simulink model "STFTDiffWindowSizes"  (R2021b)
settings: Solver=VariableStepAuto  StartTime=0.0  StopTime=2048*15/fs  RelTol=1e-3
InitFcn:
  | f = 12.288e6;
  | fs = 153.6e6;
  | N1 = 256;
  | N2 = 512;
  | N3 = 1024;
  | N4 = 2048;
  | N5 = 4096;
  | n1 = 0:N1-1;
  | n2 = 0:N2-1;
  | n3 = 0:N3-1;
  | n4 = 0:N4-1;
  | n5 = 0:N5-1;
  | Hamming1 = 0.54 - 0.46 * cos(2*pi*n1/N1);
  | Hamming2 = 0.54 - 0.46 * cos(2*pi*n2/N2);
  | Hamming3 = 0.54 - 0.46 * cos(2*pi*n3/N3);
  | Hamming4 = 0.54 - 0.46 * cos(2*pi*n4/N4);
  | Hamming5 = 0.54 - 0.46 * cos(2*pi*n5/N5);
  | Hanning1 = 0.5 * (1 + cos(2*pi*n1/N1));
  | Hanning2 = 0.5 * (1 + cos(2*pi*n2/N2));
  | Hanning3 = 0.5 * (1 + cos(2*pi*n3/N3));
  | Hanning4 = 0.5 * (1 + cos(2*pi*n4/N4));
  | Hanning5 = 0.5 * (1 + cos(2*pi*n5/N5));
  | Norm_Ham1 = sum(Hamming1);
  | Norm_Ham2 = sum(Hamming2);
  | Norm_Ham3 = sum(Hamming3);
  | Norm_Ham4 = sum(Hamming4);
  | Norm_Ham5 = sum(Hamming5);
  | Norm_Han1 = sum(Hanning1);
  | Norm_Han2 = sum(Hanning2);
  | Norm_Han3 = sum(Hanning3);
  | Norm_Han4 = sum(Hanning4);
  | Norm_Han5 = sum(Hanning5);
undefined symbols (not defined in the file): AXI4, Lite, Norm_Ham, Norm_Han
libraries: hdlBasic x321, hdlDSPIP x10, hdlsllib x1, vmcUtilities x1
(part 1 of 3)
settings Model: Creator=yxb20126  LastModifiedBy=yxb20126

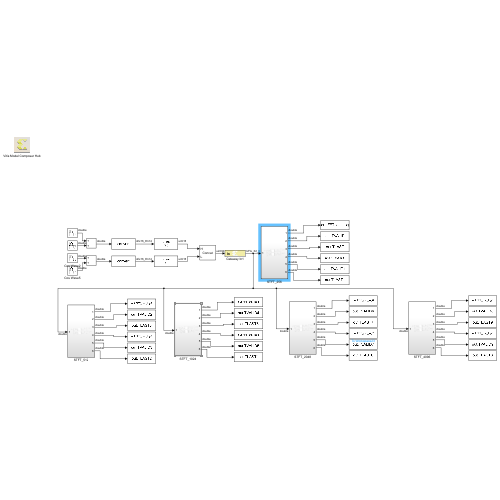
[thumbnail: Simulink's stored preview of the top-level diagram]
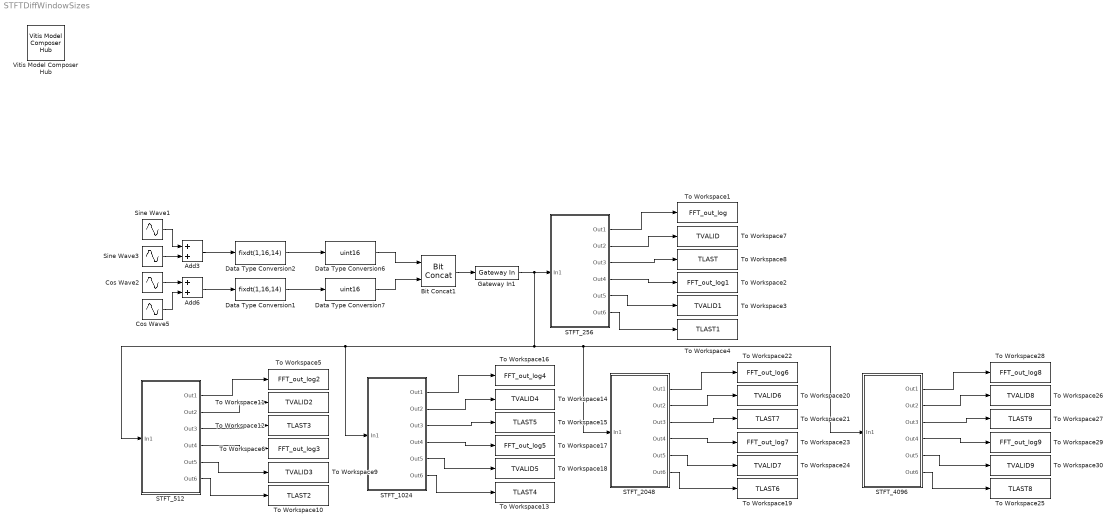
== system STFTDiffWindowSizes ==
  Add3 : Sum
  Add6 : Sum
  Bit Concat1 : hdlsllib/Logic and Bit Operations/Bit Concat  numInputs=2
  Cos Wave2 : Sin  Frequency=f*2*pi  Phase=pi/2  SampleTime=1/fs
  Cos Wave5 : Sin  Frequency=f*pi  Phase=pi/2  SampleTime=1/fs
  Data Type Conversion1 : DataTypeConversion  OutDataTypeStr=fixdt(1,16,14)  SaturateOnIntegerOverflow=on
  Data Type Conversion2 : DataTypeConversion  OutDataTypeStr=fixdt(1,16,14)  SaturateOnIntegerOverflow=on
  Data Type Conversion6 : DataTypeConversion  OutDataTypeStr=uint16  ConvertRealWorld=Stored Integer (SI)
  Data Type Conversion7 : DataTypeConversion  OutDataTypeStr=uint16  ConvertRealWorld=Stored Integer (SI)
  Gateway In1 : hdlBasic/Gateway In  gui_display_data_type=Fixed-point  arith_type=Unsigned  n_bits=32  bin_pt=0  preci_type=Single  exp_width=8  frac_width=24  rows=1  columns=1  quantization="Round  (unbiased: +/- Inf)"  overflow=Saturate  period=1/fs  UseAsADC=off  ADCChannel='1'  interface=None  automatic_assignment=on  address_offset=hex2dec('00')  intf_name=''  intf_description=''  default_value=0  timing_constraint=None  locs_specified=off  LOCs={}  io_standard={}  inherit_from_input=off  hdl_port=on  XmcBlockStatus=1  maskContainerNames=group4  block_type=gatewayin  block_config=sysgen:gateway_in_config  block_width_w=590  block_height_w=620  block_width=640  block_height=850
  STFT_1024 : Subsystem
  STFT_2048 : Subsystem
  STFT_256 : Subsystem
  STFT_4096 : Subsystem
  STFT_512 : Subsystem
  Sine Wave1 : Sin  Frequency=f*2*pi  SampleTime=1/fs
  Sine Wave3 : Sin  Frequency=f*pi  SampleTime=1/fs
  To Workspace1 : ToWorkspace  VariableName=FFT_out_log  SampleTime=-1
      settings: Save2DSignal=2-D array (concatenate along first dimension)
  To Workspace10 : ToWorkspace  VariableName=TLAST2  SampleTime=1/fs
      settings: Save2DSignal=2-D array (concatenate along first dimension)
  To Workspace11 : ToWorkspace  VariableName=TVALID2  SampleTime=1/fs
      settings: Save2DSignal=2-D array (concatenate along first dimension)
  To Workspace12 : ToWorkspace  VariableName=TLAST3  SampleTime=1/fs
      settings: Save2DSignal=2-D array (concatenate along first dimension)
  To Workspace13 : ToWorkspace  VariableName=TLAST4  SampleTime=1/fs
      settings: Save2DSignal=2-D array (concatenate along first dimension)
  To Workspace14 : ToWorkspace  VariableName=TVALID4  SampleTime=1/fs
      settings: Save2DSignal=2-D array (concatenate along first dimension)
  To Workspace15 : ToWorkspace  VariableName=TLAST5  SampleTime=1/fs
      settings: Save2DSignal=2-D array (concatenate along first dimension)
  To Workspace16 : ToWorkspace  VariableName=FFT_out_log4  SampleTime=-1
      settings: Save2DSignal=2-D array (concatenate along first dimension)
  To Workspace17 : ToWorkspace  VariableName=FFT_out_log5  SampleTime=-1
      settings: Save2DSignal=2-D array (concatenate along first dimension)
  To Workspace18 : ToWorkspace  VariableName=TVALID5  SampleTime=1/fs
      settings: Save2DSignal=2-D array (concatenate along first dimension)
  To Workspace19 : ToWorkspace  VariableName=TLAST6  SampleTime=1/fs
      settings: Save2DSignal=2-D array (concatenate along first dimension)
  To Workspace2 : ToWorkspace  VariableName=FFT_out_log1  SampleTime=-1
      settings: Save2DSignal=2-D array (concatenate along first dimension)
  To Workspace20 : ToWorkspace  VariableName=TVALID6  SampleTime=1/fs
      settings: Save2DSignal=2-D array (concatenate along first dimension)
  To Workspace21 : ToWorkspace  VariableName=TLAST7  SampleTime=1/fs
      settings: Save2DSignal=2-D array (concatenate along first dimension)
  To Workspace22 : ToWorkspace  VariableName=FFT_out_log6  SampleTime=-1
      settings: Save2DSignal=2-D array (concatenate along first dimension)
  To Workspace23 : ToWorkspace  VariableName=FFT_out_log7  SampleTime=-1
      settings: Save2DSignal=2-D array (concatenate along first dimension)
  To Workspace24 : ToWorkspace  VariableName=TVALID7  SampleTime=1/fs
      settings: Save2DSignal=2-D array (concatenate along first dimension)
  To Workspace25 : ToWorkspace  VariableName=TLAST8  SampleTime=1/fs
      settings: Save2DSignal=2-D array (concatenate along first dimension)
  To Workspace26 : ToWorkspace  VariableName=TVALID8  SampleTime=1/fs
      settings: Save2DSignal=2-D array (concatenate along first dimension)
  To Workspace27 : ToWorkspace  VariableName=TLAST9  SampleTime=1/fs
      settings: Save2DSignal=2-D array (concatenate along first dimension)
  To Workspace28 : ToWorkspace  VariableName=FFT_out_log8  SampleTime=-1
      settings: Save2DSignal=2-D array (concatenate along first dimension)
  To Workspace29 : ToWorkspace  VariableName=FFT_out_log9  SampleTime=-1
      settings: Save2DSignal=2-D array (concatenate along first dimension)
  To Workspace3 : ToWorkspace  VariableName=TVALID1  SampleTime=1/fs
      settings: Save2DSignal=2-D array (concatenate along first dimension)
  To Workspace30 : ToWorkspace  VariableName=TVALID9  SampleTime=1/fs
      settings: Save2DSignal=2-D array (concatenate along first dimension)
  To Workspace4 : ToWorkspace  VariableName=TLAST1  SampleTime=1/fs
      settings: Save2DSignal=2-D array (concatenate along first dimension)
  To Workspace5 : ToWorkspace  VariableName=FFT_out_log2  SampleTime=-1
      settings: Save2DSignal=2-D array (concatenate along first dimension)
  To Workspace6 : ToWorkspace  VariableName=FFT_out_log3  SampleTime=-1
      settings: Save2DSignal=2-D array (concatenate along first dimension)
  To Workspace7 : ToWorkspace  VariableName=TVALID  SampleTime=1/fs
      settings: Save2DSignal=2-D array (concatenate along first dimension)
  To Workspace8 : ToWorkspace  VariableName=TLAST  SampleTime=1/fs
      settings: Save2DSignal=2-D array (concatenate along first dimension)
  To Workspace9 : ToWorkspace  VariableName=TVALID3  SampleTime=1/fs
      settings: Save2DSignal=2-D array (concatenate along first dimension)
  Vitis Model Composer Hub : vmcUtilities/Vitis Model Composer Hub  Tag=genX  CodeGeneration=off  SubsystemName=<enter or select subsystem name>  TargetDirectory=./code  ExportType=HLS C++ code  IpVendor=xilinx.com  IpLibrary=hls  IpVersion=1.0  IpHWLanguage=Verilog  AieCompilerOptions={}  CreateTestbench=off  TestbenchStackSize=10  RunAieSim=off  AieSimTimeout=50000  RunAieSimProfiling=off  LaunchVitisAnalyzer=off  PlotOutput=off  RunX86Sim=off  X86SimTimeout=10  GenHwImage=off  PlatformType=Not Specified  HwSystemType=Baremetal  HwValidationTarget=hw  ProjDevice=xczu48dr-ffvg1517-2-e  ProjDevicePart=xczu48dr-ffvg1517-2-e  SamplePeriod=-1  ClockFrequency=200  DataPathParallelism=1  xilinxfamily=zynquplusRFSOC  part=xczu48dr  speed=-2-e  package=ffvg1517  directory=./netlist  testbench=off  incr_netlist=off  synthesis_tool=Vivado  clock_wrapper=Clock Enables  dbl_ovrd=According to Block Masks  dcm_input_clock_period=10  sysclk_period=(1/fs)*10e9  simulink_period=1/fs  eval_field=0
  wires:
  Data Type Conversion1/1 -> Data Type Conversion7/1
  Data Type Conversion2/1 -> Data Type Conversion6/1
  Data Type Conversion6/1 -> Bit Concat1/1
  Bit Concat1/1 -> Gateway In1/1
  Add3/1 -> Data Type Conversion2/1
  Add6/1 -> Data Type Conversion1/1
  Data Type Conversion7/1 -> Bit Concat1/2
  Gateway In1/1 -> STFT_1024/1(In1), STFT_512/1(In1), STFT_2048/1(In1), STFT_4096/1(In1), STFT_256/1(In1)
  Cos Wave2/1 -> Add6/1
  Sine Wave1/1 -> Add3/1
  Cos Wave5/1 -> Add6/2
  Sine Wave3/1 -> Add3/2
  STFT_256/1(Out1) -> To Workspace1/1
  STFT_256/2(Out2) -> To Workspace7/1
  STFT_256/3(Out3) -> To Workspace8/1
  STFT_256/4(Out4) -> To Workspace2/1
  STFT_256/5(Out5) -> To Workspace3/1
  STFT_256/6(Out6) -> To Workspace4/1
  STFT_512/6(Out6) -> To Workspace10/1
  STFT_512/5(Out5) -> To Workspace9/1
  STFT_512/4(Out4) -> To Workspace6/1
  STFT_512/3(Out3) -> To Workspace12/1
  STFT_512/2(Out2) -> To Workspace11/1
  STFT_512/1(Out1) -> To Workspace5/1
  STFT_1024/1(Out1) -> To Workspace16/1
  STFT_1024/2(Out2) -> To Workspace14/1
  STFT_1024/3(Out3) -> To Workspace15/1
  STFT_1024/4(Out4) -> To Workspace17/1
  STFT_1024/5(Out5) -> To Workspace18/1
  STFT_1024/6(Out6) -> To Workspace13/1
  STFT_2048/6(Out6) -> To Workspace19/1
  STFT_2048/5(Out5) -> To Workspace24/1
  STFT_2048/4(Out4) -> To Workspace23/1
  STFT_2048/3(Out3) -> To Workspace21/1
  STFT_2048/2(Out2) -> To Workspace20/1
  STFT_2048/1(Out1) -> To Workspace22/1
  STFT_4096/1(Out1) -> To Workspace28/1
  STFT_4096/2(Out2) -> To Workspace26/1
  STFT_4096/3(Out3) -> To Workspace27/1
  STFT_4096/4(Out4) -> To Workspace29/1
  STFT_4096/5(Out5) -> To Workspace30/1
  STFT_4096/6(Out6) -> To Workspace25/1

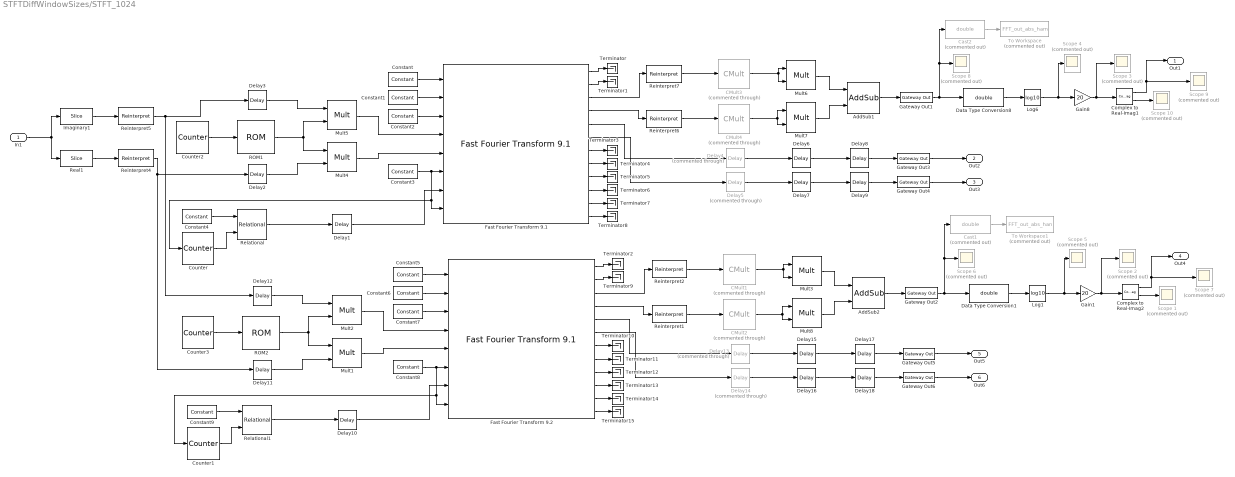
== system STFTDiffWindowSizes/STFT_1024 ==
  In1 : Inport
  AddSub1 : hdlBasic/AddSub  mode=Addition  use_carryin=off  use_carryout=off  en=off  latency=1  precision=User Defined  arith_type=Unsigned  n_bits=32  bin_pt=30  quantization=Truncate  overflow=Saturate  use_behavioral_HDL=off  hw_selection=Fabric  pipelined=off  XmcBlockStatus=1  maskContainerNames=tabcontainer1  block_type=addsub  block_config=sysgen:Addsub_config
  AddSub2 : hdlBasic/AddSub  mode=Addition  use_carryin=off  use_carryout=off  en=off  latency=1  precision=User Defined  arith_type=Unsigned  n_bits=32  bin_pt=30  quantization=Truncate  overflow=Saturate  use_behavioral_HDL=off  hw_selection=Fabric  pipelined=off  XmcBlockStatus=1  maskContainerNames=tabcontainer1  block_type=addsub  block_config=sysgen:Addsub_config
  CMult1 : hdlBasic/CMult  Commented=through  const=1/Norm_Han  gui_display_data_type=Fixed-point  const_n_bits=32  const_bin_pt=31  float_type=Single  exp_bits=8  fraction_bits=24  en=off  latency=3  precision=User Defined  arith_type=Unsigned  n_bits=32  bin_pt=31  quantization=Truncate  overflow=Saturate  use_behavioral_HDL=off  mem_type=Distributed RAM  pipeline=off  XmcBlockStatus=1  maskContainerNames=tabcontainer1  block_type=cmult  block_config=sysgen:CMult_config
      settings: infoedit=[]
  CMult2 : hdlBasic/CMult  Commented=through  const=1/Norm_Han  gui_display_data_type=Fixed-point  const_n_bits=32  const_bin_pt=31  float_type=Single  exp_bits=8  fraction_bits=24  en=off  latency=3  precision=User Defined  arith_type=Unsigned  n_bits=32  bin_pt=31  quantization=Truncate  overflow=Saturate  use_behavioral_HDL=off  mem_type=Distributed RAM  pipeline=off  XmcBlockStatus=1  maskContainerNames=tabcontainer1  block_type=cmult  block_config=sysgen:CMult_config
      settings: infoedit=[]
  CMult3 : hdlBasic/CMult  Commented=through  const=1/Norm_Ham  gui_display_data_type=Fixed-point  const_n_bits=32  const_bin_pt=31  float_type=Single  exp_bits=8  fraction_bits=24  en=off  latency=3  precision=User Defined  arith_type=Unsigned  n_bits=32  bin_pt=31  quantization=Truncate  overflow=Saturate  use_behavioral_HDL=off  mem_type=Distributed RAM  pipeline=off  XmcBlockStatus=1  maskContainerNames=tabcontainer1  block_type=cmult  block_config=sysgen:CMult_config
      settings: infoedit=[]
  CMult4 : hdlBasic/CMult  Commented=through  const=1/Norm_Ham  gui_display_data_type=Fixed-point  const_n_bits=32  const_bin_pt=31  float_type=Single  exp_bits=8  fraction_bits=24  en=off  latency=3  precision=User Defined  arith_type=Unsigned  n_bits=32  bin_pt=31  quantization=Truncate  overflow=Saturate  use_behavioral_HDL=off  mem_type=Distributed RAM  pipeline=off  XmcBlockStatus=1  maskContainerNames=tabcontainer1  block_type=cmult  block_config=sysgen:CMult_config
      settings: infoedit=[]
  Cast1 : DataTypeConversion  Commented=on  OutDataTypeStr=double
  Cast2 : DataTypeConversion  Commented=on  OutDataTypeStr=double
  Complex to Real-Imag1 : ComplexToRealImag
  Complex to Real-Imag2 : ComplexToRealImag
  Constant : hdlBasic/Constant  const=0  gui_display_data_type=Fixed-point  arith_type=Unsigned  n_bits=10  bin_pt=0  preci_type=Single  exp_width=8  frac_width=24  explicit_period=on  period=1/fs  XmcBlockStatus=1  maskContainerNames=tabcontainer1  block_type=constant  block_config=sysgen:Constant_config
  Constant1 : hdlBasic/Constant  const=0  gui_display_data_type=Fixed-point  arith_type=Unsigned  n_bits=1  bin_pt=0  preci_type=Single  exp_width=8  frac_width=24  explicit_period=on  period=1/fs  XmcBlockStatus=1  maskContainerNames=tabcontainer1  block_type=constant  block_config=sysgen:Constant_config
  Constant2 : hdlBasic/Constant  const=0  gui_display_data_type=Boolean  arith_type=Boolean  n_bits=1  bin_pt=0  preci_type=Single  exp_width=8  frac_width=24  explicit_period=on  period=1/fs  XmcBlockStatus=1  maskContainerNames=tabcontainer1  block_type=constant  block_config=sysgen:Constant_config
  Constant3 : hdlBasic/Constant  const=1  gui_display_data_type=Boolean  arith_type=Boolean  n_bits=1  bin_pt=0  preci_type=Single  exp_width=8  frac_width=24  explicit_period=on  period=1/fs  XmcBlockStatus=1  maskContainerNames=tabcontainer1  block_type=constant  block_config=sysgen:Constant_config
  Constant4 : hdlBasic/Constant  const=N3-1  gui_display_data_type=Fixed-point  arith_type=Unsigned  n_bits=10  bin_pt=0  preci_type=Single  exp_width=8  frac_width=24  explicit_period=on  period=1/fs  XmcBlockStatus=1  maskContainerNames=tabcontainer1  block_type=constant  block_config=sysgen:Constant_config
  Constant5 : hdlBasic/Constant  const=0  gui_display_data_type=Fixed-point  arith_type=Unsigned  n_bits=10  bin_pt=0  preci_type=Single  exp_width=8  frac_width=24  explicit_period=on  period=1/fs  XmcBlockStatus=1  maskContainerNames=tabcontainer1  block_type=constant  block_config=sysgen:Constant_config
  Constant6 : hdlBasic/Constant  const=0  gui_display_data_type=Fixed-point  arith_type=Unsigned  n_bits=1  bin_pt=0  preci_type=Single  exp_width=8  frac_width=24  explicit_period=on  period=1/fs  XmcBlockStatus=1  maskContainerNames=tabcontainer1  block_type=constant  block_config=sysgen:Constant_config
  Constant7 : hdlBasic/Constant  const=0  gui_display_data_type=Boolean  arith_type=Boolean  n_bits=1  bin_pt=0  preci_type=Single  exp_width=8  frac_width=24  explicit_period=on  period=1/fs  XmcBlockStatus=1  maskContainerNames=tabcontainer1  block_type=constant  block_config=sysgen:Constant_config
  Constant8 : hdlBasic/Constant  const=1  gui_display_data_type=Boolean  arith_type=Boolean  n_bits=1  bin_pt=0  preci_type=Single  exp_width=8  frac_width=24  explicit_period=on  period=1/fs  XmcBlockStatus=1  maskContainerNames=tabcontainer1  block_type=constant  block_config=sysgen:Constant_config
  Constant9 : hdlBasic/Constant  const=N3-1  gui_display_data_type=Fixed-point  arith_type=Unsigned  n_bits=10  bin_pt=0  preci_type=Single  exp_width=8  frac_width=24  explicit_period=on  period=1/fs  XmcBlockStatus=1  maskContainerNames=tabcontainer1  block_type=constant  block_config=sysgen:Constant_config
  Counter : hdlBasic/Counter  cnt_type=Count limited  cnt_to=N1-1  operation=Up  start_count=0  cnt_by_val=1  arith_type=Unsigned  n_bits=8  bin_pt=0  load_pin=off  rst=off  en=on  explicit_period=Explicit  period=1/fs  use_behavioral_HDL=off  implementation=Fabric  XmcBlockStatus=1  maskContainerNames=group1  block_type=counter  block_config=sysgen:Counter_config
  Counter1 : hdlBasic/Counter  cnt_type=Count limited  cnt_to=N3-1  operation=Up  start_count=0  cnt_by_val=1  arith_type=Unsigned  n_bits=10  bin_pt=0  load_pin=off  rst=off  en=on  explicit_period=Explicit  period=1/fs  use_behavioral_HDL=off  implementation=Fabric  XmcBlockStatus=1  maskContainerNames=group1  block_type=counter  block_config=sysgen:Counter_config
  Counter2 : hdlBasic/Counter  cnt_type=Count limited  cnt_to=N3-1  operation=Up  start_count=0  cnt_by_val=1  arith_type=Unsigned  n_bits=10  bin_pt=0  load_pin=off  rst=off  en=off  explicit_period=Explicit  period=1/fs  use_behavioral_HDL=off  implementation=Fabric  XmcBlockStatus=1  maskContainerNames=group1  block_type=counter  block_config=sysgen:Counter_config
  Counter3 : hdlBasic/Counter  cnt_type=Count limited  cnt_to=N3-1  operation=Up  start_count=0  cnt_by_val=1  arith_type=Unsigned  n_bits=10  bin_pt=0  load_pin=off  rst=off  en=off  explicit_period=Explicit  period=1/fs  use_behavioral_HDL=off  implementation=Fabric  XmcBlockStatus=1  maskContainerNames=group1  block_type=counter  block_config=sysgen:Counter_config
  Data Type Conversion1 : DataTypeConversion  OutDataTypeStr=double  SaturateOnIntegerOverflow=on
  Data Type Conversion8 : DataTypeConversion  OutDataTypeStr=double  SaturateOnIntegerOverflow=on
  Delay{1,6..7,10,15..16} (6 alike) : hdlBasic/Delay  rst=off  en=off  latency=3  reg_retiming=off  XmcBlockStatus=1  maskContainerNames=group1  block_type=delay  block_config=sysgen:Delay_config
  Delay{2..3,8..9,11..12,17..18} (8 alike) : hdlBasic/Delay  rst=off  en=off  latency=1  reg_retiming=off  XmcBlockStatus=1  maskContainerNames=group1  block_type=delay  block_config=sysgen:Delay_config
  Delay{4..5,13..14} (4 alike) : hdlBasic/Delay  Commented=through  rst=off  en=off  latency=3  reg_retiming=off  XmcBlockStatus=1  maskContainerNames=group1  block_type=delay  block_config=sysgen:Delay_config
  Fast Fourier Transform 9.1 : hdlDSPIP/Fast Fourier Transform 9.1   transform_length=1024  target_clock_frequency=200  target_data_throughput=50  implementation_options=pipelined_streaming_io  run_time_configurable_transform_length=off  phase_factor_width=16  scaling_options=scaled  rounding_modes=truncation  aclken=off  aresetn=off  output_ordering=natural_order  cyclic_prefix_insertion=off  throttle_scheme=nonrealtime  xk_index=off  ovflo=off  trim_axipin_name=on  memory_options_data=block_ram  memory_options_phase_factors=block_ram  number_of_stages_using_block_ram_for_data_and_phase_factors=5  memory_options_reorder=block_ram  memory_options_hybrid=off  complex_mult_type=use_mults_resources  butterfly_type=use_luts  simulation_type=hybrid_sim  simulation_model=sysgen:xfftv9_cmodel  data_path_portlist={ 's_axis_data_tdata', 'm_axis_data_tdata', 'm_axis_status_tdata', 'event_fft_overflow' }  channels=1  input_ordering=natural_order  input_width=16  ip_name=Fast Fourier Transform  ip_version=9.1  dsptool_ready=true  ipcore_usecache=true  ipcore_useipmodelcache=true  wrapper_available=true  port_translation_map={ 'aclken' => 'en', 'aresetn' => 'rst'}  data_format=fixed_point  XmcBlockStatus=1  maskContainerNames=tabcontainer1  block_type=xfft_v9_1  block_config=sysgen:rodinimport_config
  Fast Fourier Transform 9.2 : hdlDSPIP/Fast Fourier Transform 9.1   transform_length=1024  target_clock_frequency=200  target_data_throughput=50  implementation_options=pipelined_streaming_io  run_time_configurable_transform_length=off  phase_factor_width=16  scaling_options=scaled  rounding_modes=truncation  aclken=off  aresetn=off  output_ordering=natural_order  cyclic_prefix_insertion=off  throttle_scheme=nonrealtime  xk_index=off  ovflo=off  trim_axipin_name=on  memory_options_data=block_ram  memory_options_phase_factors=block_ram  number_of_stages_using_block_ram_for_data_and_phase_factors=5  memory_options_reorder=block_ram  memory_options_hybrid=off  complex_mult_type=use_mults_resources  butterfly_type=use_luts  simulation_type=hybrid_sim  simulation_model=sysgen:xfftv9_cmodel  data_path_portlist={ 's_axis_data_tdata', 'm_axis_data_tdata', 'm_axis_status_tdata', 'event_fft_overflow' }  channels=1  input_ordering=natural_order  input_width=16  ip_name=Fast Fourier Transform  ip_version=9.1  dsptool_ready=true  ipcore_usecache=true  ipcore_useipmodelcache=true  wrapper_available=true  port_translation_map={ 'aclken' => 'en', 'aresetn' => 'rst'}  data_format=fixed_point  XmcBlockStatus=1  maskContainerNames=tabcontainer1  block_type=xfft_v9_1  block_config=sysgen:rodinimport_config
  Gain1 : Gain  Gain=20
  Gain8 : Gain  Gain=20
  Gateway Out1 : hdlBasic/Gateway Out  inherit_from_input=on  hdl_port=on  rows=1  columns=1  UseAsDAC=off  DACChannel='1'  interface=AXI4-Lite  automatic_assignment=on  address_offset=hex2dec('00')  intf_name=''  intf_description=''  timing_constraint=None  locs_specified=off  LOCs={}  io_standard={}  XmcBlockStatus=1  maskContainerNames=group4  block_type=gatewayout  block_config=sysgen:gateway_out_config  block_width_w=590  block_height_w=620  block_width=620  block_height=750
  Gateway Out2 : hdlBasic/Gateway Out  inherit_from_input=on  hdl_port=on  rows=1  columns=1  UseAsDAC=off  DACChannel='1'  interface=AXI4-Lite  automatic_assignment=on  address_offset=hex2dec('00')  intf_name=''  intf_description=''  timing_constraint=None  locs_specified=off  LOCs={}  io_standard={}  XmcBlockStatus=1  maskContainerNames=group4  block_type=gatewayout  block_config=sysgen:gateway_out_config  block_width_w=590  block_height_w=620  block_width=620  block_height=750
  Gateway Out{3..6} (4 alike) : hdlBasic/Gateway Out  inherit_from_input=off  hdl_port=on  rows=1  columns=1  UseAsDAC=off  DACChannel='1'  interface=AXI4-Lite  automatic_assignment=on  address_offset=hex2dec('00')  intf_name=''  intf_description=''  timing_constraint=None  locs_specified=off  LOCs={}  io_standard={}  XmcBlockStatus=1  maskContainerNames=group4  block_type=gatewayout  block_config=sysgen:gateway_out_config  block_width_w=590  block_height_w=620  block_width=620  block_height=750
  Imaginary1 : hdlBasic/Slice  nbits=16  boolean_output=off  mode=Two Bit Locations  bit1=31  base1=LSB of Input  bit0=16  base0=LSB of Input  XmcBlockStatus=1  maskContainerNames=group1  block_type=slice  block_config=sysgen:Slice_config
  Log1 : Math  Operator=log10  OutputSignalType=complex  SaturateOnIntegerOverflow=on
  Log6 : Math  Operator=log10  OutputSignalType=complex  SaturateOnIntegerOverflow=on
  Mult{1..2,4..5} (4 alike) : hdlBasic/Mult  precision=User Defined  arith_type="Signed  (2's comp)"  n_bits=16  bin_pt=15  quantization=Truncate  overflow=Saturate  en=off  latency=3  use_behavioral_HDL=off  opt=Speed  use_embedded=on  optimum_pipeline=off  pipeline=on  use_rpm=on  placement_style=Triangular  XmcBlockStatus=1  maskContainerNames=group1  block_type=mult  block_config=sysgen:Mult_config
  Mult{3,6..8} (4 alike) : hdlBasic/Mult  precision=User Defined  arith_type=Unsigned  n_bits=32  bin_pt=31  quantization=Truncate  overflow=Saturate  en=off  latency=3  use_behavioral_HDL=off  opt=Speed  use_embedded=on  optimum_pipeline=off  pipeline=on  use_rpm=on  placement_style=Triangular  XmcBlockStatus=1  maskContainerNames=group1  block_type=mult  block_config=sysgen:Mult_config
  ROM1 : hdlBasic/ROM  depth=N3  initVector=Hamming3  distributed_mem=Block RAM  rst=off  init_reg=0  en=off  latency=1  gui_display_data_type=Fixed-point  arith_type=Unsigned  n_bits=16  bin_pt=15  preci_type=Single  exp_width=8  frac_width=24  optimize=Area  use_rpm=on  simulation_type=fast_sim  XmcBlockStatus=1  maskContainerNames=tabcontainer1  block_type=sprom  block_config=sysgen:SPROM_config
  ROM2 : hdlBasic/ROM  depth=N3  initVector=Hanning3  distributed_mem=Block RAM  rst=off  init_reg=0  en=off  latency=1  gui_display_data_type=Fixed-point  arith_type=Unsigned  n_bits=16  bin_pt=15  preci_type=Single  exp_width=8  frac_width=24  optimize=Area  use_rpm=on  simulation_type=fast_sim  XmcBlockStatus=1  maskContainerNames=tabcontainer1  block_type=sprom  block_config=sysgen:SPROM_config
  Real1 : hdlBasic/Slice  nbits=16  boolean_output=off  mode=Two Bit Locations  bit1=15  base1=LSB of Input  bit0=0  base0=LSB of Input  XmcBlockStatus=1  maskContainerNames=group1  block_type=slice  block_config=sysgen:Slice_config
  Reinterpret{1..2,6..7} (4 alike) : hdlBasic/Reinterpret  force_arith_type=on  arith_type="Signed  (2's comp)"  force_bin_pt=off  bin_pt=31  XmcBlockStatus=1  maskContainerNames=group1  block_type=reinterpret  block_config=sysgen:Reinterpret_config
  Reinterpret4 : hdlBasic/Reinterpret  force_arith_type=on  arith_type="Signed  (2's comp)"  force_bin_pt=on  bin_pt=14  XmcBlockStatus=1  maskContainerNames=group1  block_type=reinterpret  block_config=sysgen:Reinterpret_config
  Reinterpret5 : hdlBasic/Reinterpret  force_arith_type=on  arith_type="Signed  (2's comp)"  force_bin_pt=on  bin_pt=14  XmcBlockStatus=1  maskContainerNames=group1  block_type=reinterpret  block_config=sysgen:Reinterpret_config
  Relational : hdlBasic/Relational  mode=a=b  op_type=Bool  en=off  latency=1  XmcBlockStatus=1  maskContainerNames=tabcontainer1  block_type=relational  block_config=sysgen:Relational_config
  Relational1 : hdlBasic/Relational  mode=a=b  op_type=Bool  en=off  latency=1  XmcBlockStatus=1  maskContainerNames=tabcontainer1  block_type=relational  block_config=sysgen:Relational_config
  Scope {1..10} (10 alike) : Scope  Commented=on
  Terminator{,1..15} (16 alike) : Terminator
  To Workspace : ToWorkspace  Commented=on  VariableName=FFT_out_abs_ham  SampleTime=-1
      settings: Save2DSignal=2-D array (concatenate along first dimension)
  To Workspace1 : ToWorkspace  Commented=on  VariableName=FFT_out_abs_han  SampleTime=-1
      settings: Save2DSignal=2-D array (concatenate along first dimension)
  Out1 : Outport
  Out2 : Outport  Port=2
  Out3 : Outport  Port=3
  Out4 : Outport  Port=4
  Out5 : Outport  Port=5
  Out6 : Outport  Port=6
  wires:
  Constant2/1 -> Fast Fourier Transform 9.1/3
  Fast Fourier Transform 9.1/5 -> Delay4/1
  Delay8/1 -> Gateway Out3/1
  Constant3/1 -> Fast Fourier Transform 9.1/6, Fast Fourier Transform 9.1/8, Counter/1
  Delay4/1 -> Delay6/1
  Delay7/1 -> Delay9/1
  Delay2/1 -> Mult4/2
  ROM1/1 -> Mult5/2, Mult4/1
  Delay6/1 -> Delay8/1
  Fast Fourier Transform 9.1/3 -> Reinterpret7/1
  Gateway Out1/1 -> Cast2/1, Scope 8/1, Data Type Conversion8/1
  Constant1/1 -> Fast Fourier Transform 9.1/2
  Fast Fourier Transform 9.1/7 -> Terminator3/1
  Fast Fourier Transform 9.1/1 -> Terminator/1
  Fast Fourier Transform 9.1/10 -> Terminator6/1
  Fast Fourier Transform 9.1/12 -> Terminator8/1
  Fast Fourier Transform 9.1/6 -> Delay5/1
  Imaginary1/1 -> Reinterpret5/1
  Constant/1 -> Fast Fourier Transform 9.1/1
  Fast Fourier Transform 9.1/2 -> Terminator1/1
  Delay1/1 -> Fast Fourier Transform 9.1/7
  In1/1 -> Real1/1, Imaginary1/1
  Reinterpret6/1 -> CMult4/1
  Gateway Out3/1 -> Out2/1
  AddSub1/1 -> Gateway Out1/1
  Gateway Out4/1 -> Out3/1
  Fast Fourier Transform 9.1/4 -> Reinterpret6/1
  Delay5/1 -> Delay7/1
  CMult3/1 -> Mult6/1, Mult6/2
  Fast Fourier Transform 9.1/11 -> Terminator7/1
  CMult4/1 -> Mult7/1, Mult7/2
  Mult4/1 -> Fast Fourier Transform 9.1/5
  Complex to Real-Imag1/1 -> Out1/1, Scope 9/1
  Counter/1 -> Relational/2
  Gain8/1 -> Scope 3/1, Complex to Real-Imag1/1
  Log6/1 -> Scope 4/1, Gain8/1
  Mult7/1 -> AddSub1/2
  Reinterpret7/1 -> CMult3/1
  Fast Fourier Transform 9.1/8 -> Terminator4/1
  Complex to Real-Imag1/2 -> Scope 10/1
  Real1/1 -> Reinterpret4/1
  Constant4/1 -> Relational/1
  Data Type Conversion8/1 -> Log6/1
  Counter2/1 -> ROM1/1
  Mult5/1 -> Fast Fourier Transform 9.1/4
  Relational/1 -> Delay1/1
  Mult6/1 -> AddSub1/1
  Cast2/1 -> To Workspace/1
  Delay9/1 -> Gateway Out4/1
  Delay3/1 -> Mult5/1
  Fast Fourier Transform 9.1/9 -> Terminator5/1
  Fast Fourier Transform 9.2/9 -> Terminator12/1
  Delay12/1 -> Mult2/1
  Delay18/1 -> Gateway Out6/1
  Cast1/1 -> To Workspace1/1
  Mult3/1 -> AddSub2/1
  Relational1/1 -> Delay10/1
  Mult2/1 -> Fast Fourier Transform 9.2/4
  Counter3/1 -> ROM2/1
  Data Type Conversion1/1 -> Log1/1
  Constant9/1 -> Relational1/1
  Complex to Real-Imag2/2 -> Scope 1/1
  Fast Fourier Transform 9.2/8 -> Terminator11/1
  Reinterpret2/1 -> CMult1/1
  Reinterpret4/1 -> Delay11/1, Delay2/1
  Mult8/1 -> AddSub2/2
  Log1/1 -> Gain1/1, Scope 5/1
  Gain1/1 -> Complex to Real-Imag2/1, Scope 2/1
  Counter1/1 -> Relational1/2
  Complex to Real-Imag2/1 -> Scope 7/1, Out4/1
  Mult1/1 -> Fast Fourier Transform 9.2/5
  CMult2/1 -> Mult8/2, Mult8/1
  Reinterpret5/1 -> Delay12/1, Delay3/1
  Fast Fourier Transform 9.2/11 -> Terminator14/1
  CMult1/1 -> Mult3/2, Mult3/1
  Delay14/1 -> Delay16/1
  Fast Fourier Transform 9.2/4 -> Reinterpret1/1
  Gateway Out6/1 -> Out6/1
  AddSub2/1 -> Gateway Out2/1
  Gateway Out5/1 -> Out5/1
  Reinterpret1/1 -> CMult2/1
  Delay10/1 -> Fast Fourier Transform 9.2/7
  Fast Fourier Transform 9.2/2 -> Terminator9/1
  Constant5/1 -> Fast Fourier Transform 9.2/1
  Fast Fourier Transform 9.2/6 -> Delay14/1
  Fast Fourier Transform 9.2/12 -> Terminator15/1
  Fast Fourier Transform 9.2/10 -> Terminator13/1
  Fast Fourier Transform 9.2/1 -> Terminator2/1
  Fast Fourier Transform 9.2/7 -> Terminator10/1
  Constant6/1 -> Fast Fourier Transform 9.2/2
  Gateway Out2/1 -> Data Type Conversion1/1, Scope 6/1, Cast1/1
  Fast Fourier Transform 9.2/3 -> Reinterpret2/1
  Delay15/1 -> Delay17/1
  ROM2/1 -> Mult1/1, Mult2/2
  Delay11/1 -> Mult1/2
  Delay16/1 -> Delay18/1
  Delay13/1 -> Delay15/1
  Constant8/1 -> Counter1/1, Fast Fourier Transform 9.2/8, Fast Fourier Transform 9.2/6
  Delay17/1 -> Gateway Out5/1
  Fast Fourier Transform 9.2/5 -> Delay13/1
  Constant7/1 -> Fast Fourier Transform 9.2/3
